simulink model "SFOI_LQG"  (R2024b)
settings: Solver=VariableStepAuto  StartTime=0.0  StopTime=ST  RelTol=1e-3
InitFcn:
  | % clear all
  | % close all
  | % clc
  | %
  | % % Load Modello e Parametri
  | % load("model.mat");
  | %
  | % load("Ass_autovalori.mat");
  | %
  | % double_A = double(A_lin);
  | % double_B = double(B_lin);
  | % C = [1 0 0 0 0 0; 0 0 1 0 0 0; 0 0 0 0 1 0];
  | % D = zeros(3,2);
  | % Kf = pinv(C*inv(A_closed_loop)*double_B);
  | %
  | % % Condizioni iniziali
  | % x0 = [0, 0, 0.22, 0, 0.12, 0]; % Stato iniziale
  | %
  | % % Verifica dell'osservabilità
  | % O = obsv(A_lin, C);
  | % osservabile = rank(O) == size(double_A, 1);
  | %
  | % if osservabile
  | %     disp('Il sistema è osservabile.');
  | % else
  | %     disp('Il sistema NON è osservabile.');
  | % end
  | %
  | % % Verifica dell'osservabilità
  | % Ctrb = ctrb(double_A', C');
  | % controllabile = rank(Ctrb) == size(double_A, 1);
  | %
  | % if controllabile
  | %     disp('Il sistema è controllabile.');
  | % else
  | %     disp('Il sistema NON è controllabile.');
  | % end
  | %
  | %
  | % % Poli desiderati per l'osservatore
  | % poli_osservatore = [-80 -2 -40 -1 -30 -0.5];
  | %
  | % % Calcolo del guadagno dell'osservatore L
  | % L = place(double_A', C', poli_osservatore)';
  | %
  | % % Dinamica dell'osservatore
  | % A_o = double_A - L * C; % Matrice del sistema osservatore
  | % B_o = [double_B - L * D, L]; % Matrice degli ingressi per l'osservatore
  | % C_o = eye(6); % Gli stati stimati vengono restituiti
  | % D_o = zeros(6,5); % Dimensioni appropriate per ingressi e uscite
undefined symbols (not defined in the file or in its folder): A_obs, B_obs, C, D, double_A, double_B, K, x0, xd
settings Model: Creator=raffa  LastModifiedBy=raffa
settings RTWCC: GPUComputeCapability=3.5

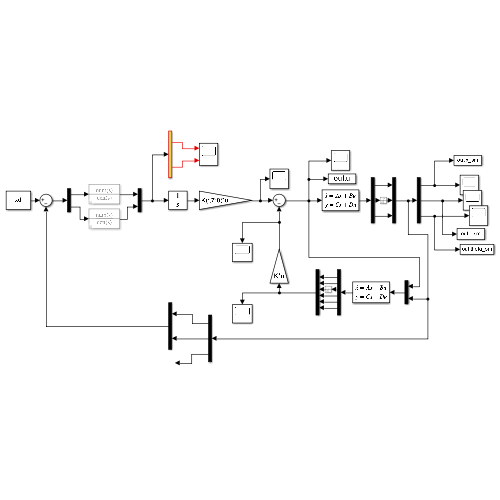
[thumbnail: Simulink's stored preview of the top-level diagram]
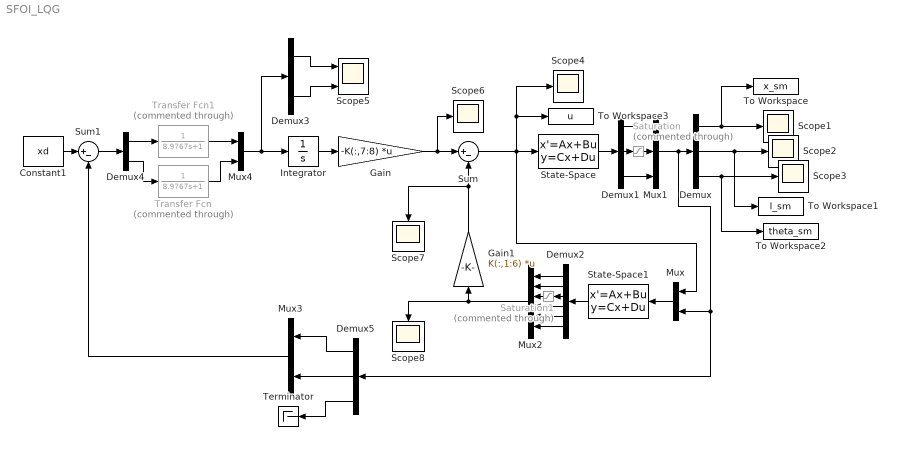
== system SFOI_LQG ==
  Constant1 : Constant  Value=xd
  Demux : Demux  Outputs=3
  Demux1 : Demux  Outputs=3
  Demux2 : Demux  Outputs=6
  Demux3 : Demux  Outputs=2
  Demux4 : Demux  Outputs=2
  Demux5 : Demux  Outputs=3
  Gain : Gain  Gain=-K(:,7:8)  Multiplication=Matrix(K*u)
  Gain1 : Gain  Gain=K(:,1:6)  Multiplication=Matrix(K*u)
  Integrator : Integrator  InitialCondition="[1 0 0 0 0 0 ; 0 0  1 0 0 0] * x0"  LowerSaturationLimit=-50
  Mux : Mux  Inputs=2
  Mux1 : Mux  Inputs=3
  Mux2 : Mux  Inputs=6
  Mux3 : Mux  Inputs=2
  Mux4 : Mux  Inputs=2
  Saturation : Saturate  Commented=through  UpperLimit=5  LowerLimit=0.1
  Saturation1 : Saturate  Commented=through  UpperLimit=5  LowerLimit=0.1
  Scope{1..4,6..8} (7 alike) : Scope
  Scope5 : Scope  NumInputPorts=2
  State-Space : StateSpace  A=double_A  B=double_B  C=C  D=D  InitialCondition=x0'
  State-Space1 : StateSpace  A=A_obs  B=B_obs  C=eye(6)  D=zeros(6,5)  InitialCondition=x0'
  Sum : Sum  Inputs=|+-
  Sum1 : Sum  Inputs=|+-
  Terminator : Terminator
  To Workspace : ToWorkspace  VariableName=x_sm  SaveFormat=Timeseries  SampleTime=-1
  To Workspace1 : ToWorkspace  VariableName=l_sm  SaveFormat=Timeseries  SampleTime=-1
  To Workspace2 : ToWorkspace  VariableName=theta_sm  SaveFormat=Timeseries  SampleTime=-1
  To Workspace3 : ToWorkspace  VariableName=u  SaveFormat=Timeseries  SampleTime=-1
  Transfer Fcn : TransferFcn  Commented=through  Denominator=[8.9767 1]
  Transfer Fcn1 : TransferFcn  Commented=through  Denominator=[8.9767 1]
  wires:
  Demux/1 -> Scope1/1, To Workspace/1
  Demux/2 -> Scope2/1, To Workspace1/1
  Demux/3 -> Scope3/1, To Workspace2/1
  Mux/1 -> State-Space1/1
  State-Space/1 -> Demux1/1
  Demux1/3 -> Mux1/3
  Demux1/2 -> Saturation/1
  Saturation/1 -> Mux1/2
  Demux1/1 -> Mux1/1
  State-Space1/1 -> Demux2/1
  Demux2/1 -> Mux2/1
  Demux2/4 -> Mux2/4
  Demux2/5 -> Mux2/5
  Demux2/6 -> Mux2/6
  Demux2/2 -> Mux2/2
  Saturation1/1 -> Mux2/3
  Demux2/3 -> Saturation1/1
  Sum/1 -> Mux/1, State-Space/1, To Workspace3/1, Scope4/1
  Demux5/2 -> Mux3/2
  Demux3/1 -> Scope5/1
  Demux5/3 -> Terminator/1
  Demux5/1 -> Mux3/1
  Demux3/2 -> Scope5/2
  Integrator/1 -> Gain/1
  Mux3/1 -> Sum1/2
  Mux1/1 -> Demux5/1, Mux/2, Demux/1
  Gain/1 -> Scope6/1, Sum/1
  Gain1/1 -> Scope7/1, Sum/2
  Mux2/1 -> Scope8/1, Gain1/1
  Constant1/1 -> Sum1/1
  Demux4/1 -> Transfer Fcn1/1
  Transfer Fcn1/1 -> Mux4/1
  Transfer Fcn/1 -> Mux4/2
  Demux4/2 -> Transfer Fcn/1
  Mux4/1 -> Demux3/1, Integrator/1
  Sum1/1 -> Demux4/1
